simulink model "kers_charge_19_6_update"  (R2019a)
settings: Solver=VariableStepAuto  StartTime=0.0  StopTime=3  RelTol=1e-3
values from neighbouring files (symbols this model uses):
  d = 0.49    [Data.m]
  Jeq_v = 120    [Data.m]
  Jf = 0.026    [Data.m]
  tau_max = 2.5    [Data.m]
  tau_min = 0.4    [Data.m]
  tau_trasm = 62.8    [Data.m]
  Tmax2 = -3675    [Data.m]
  wf_max = 60000/9.55    (= 6282.72251309)    [Data.m]
undefined symbols (not defined in the file or in its folder): Rw
settings Model: Creator=andre  LastModifiedBy=Federico Kieffer

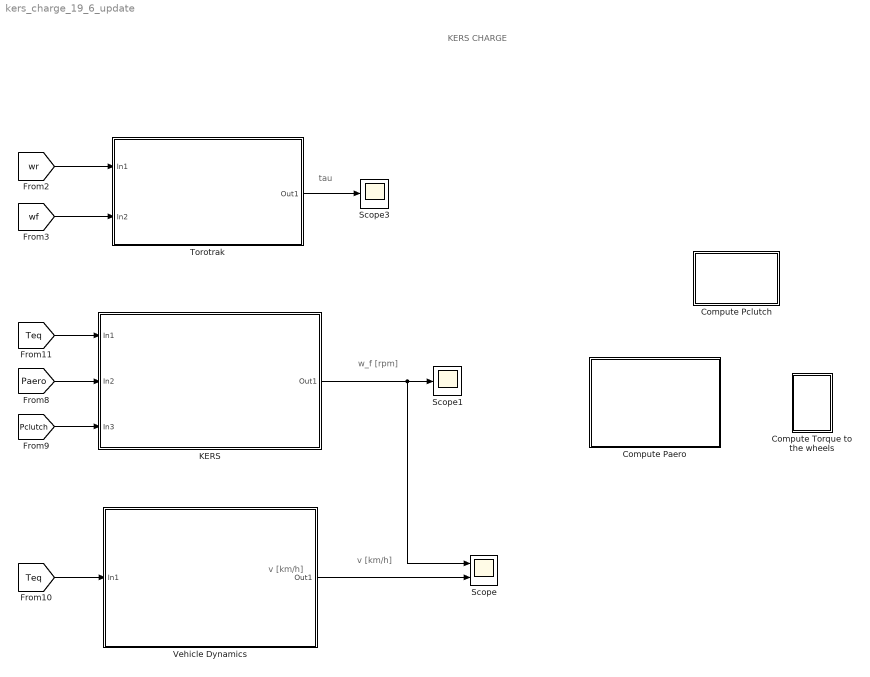
== system kers_charge_19_6_update ==
  note: KERS CHARGE
  note: v [km/h]
  note: w_f [rpm]
  note: v [km/h]
  note: tau
  Compute Paero : Subsystem
  Compute Pclutch : Subsystem
  Compute Torque to the wheels : Subsystem
  KERS : Subsystem
      mask Display: image('KERS.jpg'); % Use "Edit Image" on toolstrip to change.
  Scope : Scope  NumInputPorts=2
  Scope1 : Scope
  Scope3 : Scope
  Torotrak : Subsystem
      mask Display: image('Torotrak.jpg'); % Use "Edit Image" on toolstrip to change.
  Vehicle Dynamics : Subsystem
      mask Display: image('Ferrari.jpg'); % Use "Edit Image" on toolstrip to change.
  wires:
  [wr] -> Torotrak/1(In1)
  [wf] -> Torotrak/2(In2)
  Torotrak/1(Out1) -> Scope3/1
  [Teq] -> Vehicle Dynamics/1(In1)
  Vehicle Dynamics/1(Out1) -> Scope/2
  [Teq] -> KERS/1(In1)
  [Paero] -> KERS/2(In2)
  [Pclutch] -> KERS/3(In3)
  KERS/1(Out1) -> Scope1/1, Scope/1

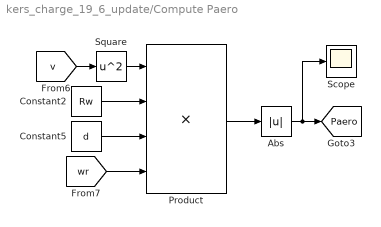
== system kers_charge_19_6_update/Compute Paero ==
  Abs : Abs  ZeroCross=off
  Constant2 : Constant  Value=Rw
  Constant5 : Constant  Value=d
  Product : Product  Inputs=4
  Scope : Scope
  Square : Math  Operator=square  SaturateOnIntegerOverflow=on
  tag scope: Paero=global
  wires:
  Square/1 -> Product/1
  Constant5/1 -> Product/3
  [wr] -> Product/4
  [v] -> Square/1
  Constant2/1 -> Product/2
  Product/1 -> Abs/1
  Abs/1 -> Scope/1, [Paero]

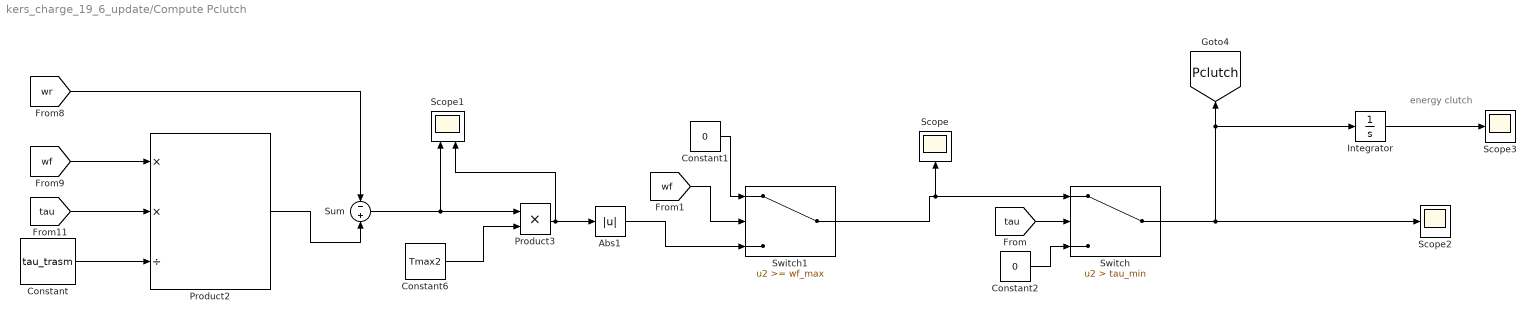
== system kers_charge_19_6_update/Compute Pclutch ==
  note: energy clutch
  Abs1 : Abs  ZeroCross=off
  Constant : Constant  Value=tau_trasm
  Constant1 : Constant  Value=0
  Constant2 : Constant  Value=0
  Constant6 : Constant  Value=Tmax2
  Integrator : Integrator
  Product2 : Product  Inputs=**/
  Product3 : Product
  Scope : Scope
  Scope1 : Scope  NumInputPorts=2
  Scope2 : Scope
  Scope3 : Scope
  Sum : Sum  Inputs=-+
  Switch : Switch  Criteria=u2 > Threshold  Threshold=tau_min
  Switch1 : Switch  Threshold=wf_max
  tag scope: Pclutch=global
  wires:
  Product2/1 -> Sum/2
  [wf] -> Product2/1
  Constant6/1 -> Product3/2
  [wr] -> Sum/1
  Constant/1 -> Product2/3
  [tau] -> Product2/2
  Sum/1 -> Product3/1, Scope1/1
  Product3/1 -> Scope1/2, Abs1/1
  Integrator/1 -> Scope3/1
  [wf] -> Switch1/2
  Constant1/1 -> Switch1/1
  Abs1/1 -> Switch1/3
  [tau] -> Switch/2
  Switch1/1 -> Switch/1, Scope/1
  Constant2/1 -> Switch/3
  Switch/1 -> Integrator/1, [Pclutch], Scope2/1

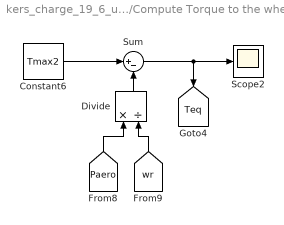
== system kers_charge_19_6_update/Compute Torque to the wheels ==
  Constant6 : Constant  Value=Tmax2
  Divide : Product  Inputs=*/
  Scope2 : Scope
  Sum : Sum  Inputs=|+-
  tag scope: Teq=global
  wires:
  Sum/1 -> [Teq], Scope2/1
  [Paero] -> Divide/1
  Constant6/1 -> Sum/1
  [wr] -> Divide/2
  Divide/1 -> Sum/2

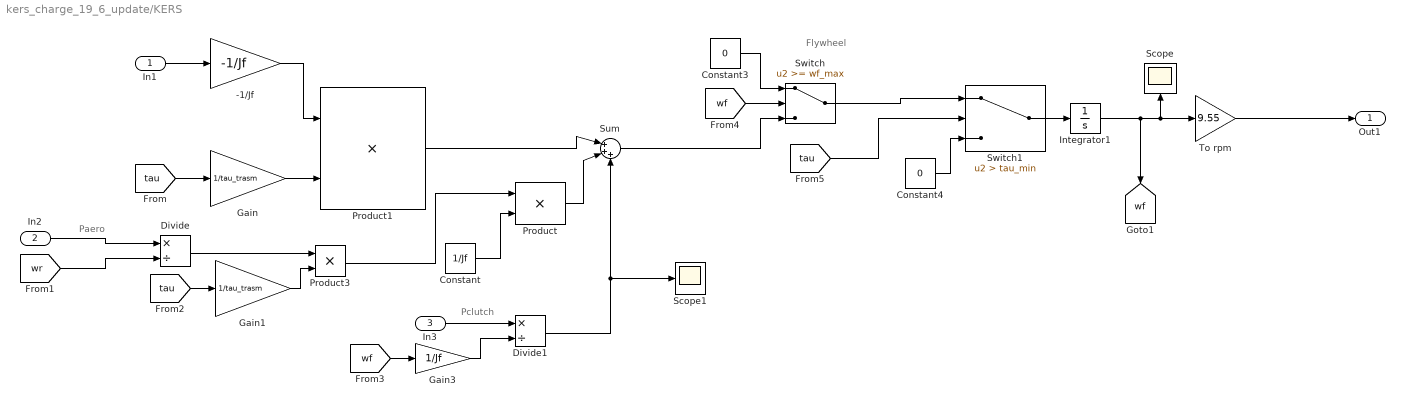
== system kers_charge_19_6_update/KERS ==
  note: Pclutch
  note: Paero
  note: Flywheel
  In1 : Inport
  In2 : Inport  Port=2
  In3 : Inport  Port=3
  -1/Jf : Gain  Gain=-1/Jf
  Constant : Constant  Value=1/Jf
  Constant3 : Constant  Value=0
  Constant4 : Constant  Value=0
  Divide : Product  Inputs=*/
  Divide1 : Product  Inputs=*/
  Gain : Gain  Gain=1/tau_trasm
  Gain1 : Gain  Gain=1/tau_trasm
  Gain3 : Gain  Gain=1/Jf
  Integrator1 : Integrator  InitialCondition=0.0001  ContinuousStateAttributes="\"omega_f\""
  Product : Product  Inputs=**
  Product1 : Product  Inputs=**
  Product3 : Product
  Scope : Scope
  Scope1 : Scope
  Sum : Sum  Inputs=|+++
  Switch : Switch  Threshold=wf_max
  Switch1 : Switch  Criteria=u2 > Threshold  Threshold=tau_min
  To rpm : Gain  Gain=9.55
  Out1 : Outport  VectorParamsAs1DForOutWhenUnconnected=on
  tag scope: wf=global
  wires:
  Sum/1 -> Switch/3
  Switch1/1 -> Integrator1/1
  -1/Jf/1 -> Product1/1
  Integrator1/1 -> Scope/1, To rpm/1, [wf]
  Constant3/1 -> Switch/1
  Switch/1 -> Switch1/1
  [wf] -> Switch/2
  Constant4/1 -> Switch1/3
  [tau] -> Switch1/2
  Product/1 -> Sum/2
  Product1/1 -> Sum/1
  To rpm/1 -> Out1/1
  In1/1 -> -1/Jf/1
  Gain/1 -> Product1/2
  [tau] -> Gain/1
  In2/1 -> Divide/1
  [wr] -> Divide/2
  Divide/1 -> Product3/1
  [tau] -> Gain1/1
  Gain1/1 -> Product3/2
  Product3/1 -> Product/1
  Constant/1 -> Product/2
  In3/1 -> Divide1/1
  [wf] -> Gain3/1
  Gain3/1 -> Divide1/2
  Divide1/1 -> Scope1/1, Sum/3

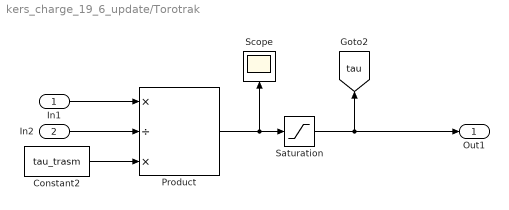
== system kers_charge_19_6_update/Torotrak ==
  In1 : Inport
  In2 : Inport  Port=2
  Constant2 : Constant  Value=tau_trasm
  Product : Product  Inputs=*/*
  Saturation : Saturate  UpperLimit=tau_max  LowerLimit=tau_min
  Scope : Scope
  Out1 : Outport  VectorParamsAs1DForOutWhenUnconnected=on
  tag scope: tau=global
  wires:
  In2/1 -> Product/2
  Constant2/1 -> Product/3
  Saturation/1 -> Out1/1, [tau]
  In1/1 -> Product/1
  Product/1 -> Scope/1, Saturation/1

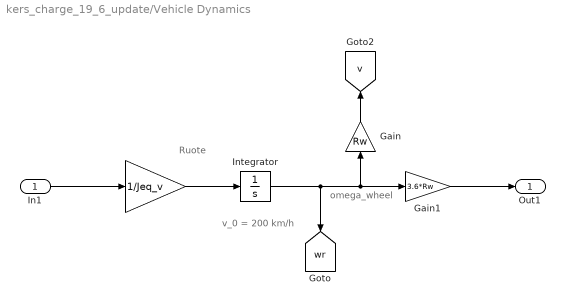
== system kers_charge_19_6_update/Vehicle Dynamics ==
  note: omega_wheel
  note: v_0 = 200 km/h
  note: Ruote
  In1 : Inport
  " " : Gain  Gain=1/Jeq_v
  Gain : Gain  Gain=Rw
  Gain1 : Gain  Gain=3.6*Rw
  Integrator : Integrator  InitialCondition=300/(3.6*Rw)  ContinuousStateAttributes="\"omega_w\""
  Out1 : Outport  VectorParamsAs1DForOutWhenUnconnected=on
  tag scope: v=global, wr=global
  wires:
  Integrator/1 -> Gain/1, Gain1/1, [wr]
  In1/1 -> " "/1
  Gain/1 -> [v]
  " "/1 -> Integrator/1
  Gain1/1 -> Out1/1
